simulink model "StabilityObserverPosition"  (R2016b)
settings: configuration reference "WheelSimConfiguration2016" (kept outside this file)
undefined symbols (not defined in the file): simulator
settings Model: Creator=At  LastModifiedBy=At
settings ConfigSetRef: SourceLocation=Base Workspace

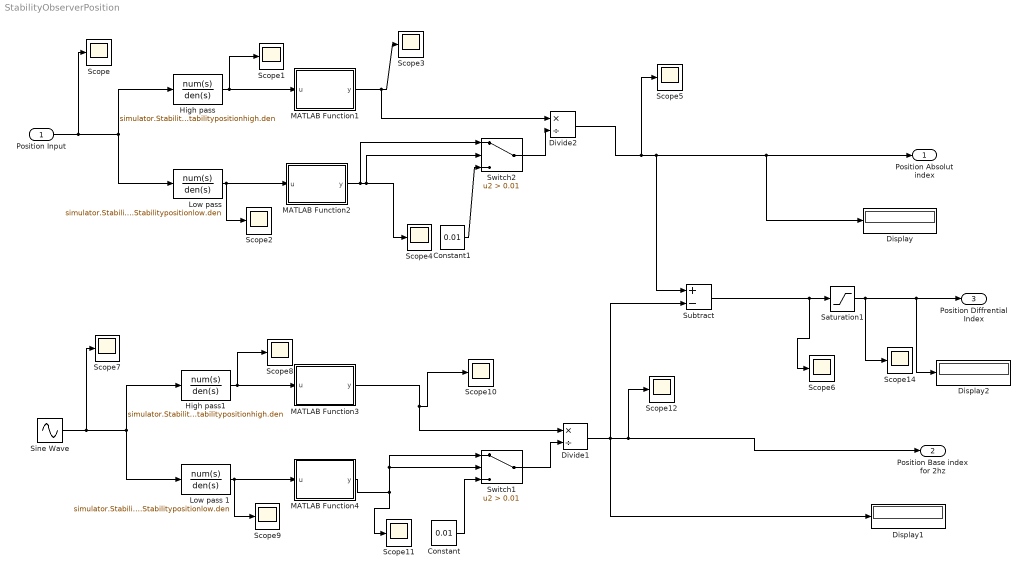
== system StabilityObserverPosition ==
  Position Input : Inport
  Constant : Constant  Value=0.01
  Constant1 : Constant  Value=0.01
  Display : Display
  Display1 : Display
  Display2 : Display
  Divide1 : Product  Inputs=*/
  Divide2 : Product  Inputs=*/
  High pass : TransferFcn  Numerator=simulator.Stabilitypositionhigh.num  Denominator=simulator.Stabilitypositionhigh.den
  High pass1 : TransferFcn  Numerator=simulator.Stabilitypositionhigh.num  Denominator=simulator.Stabilitypositionhigh.den
  "Low pass " : TransferFcn  Numerator=simulator.Stabilitypositionlow.num  Denominator=simulator.Stabilitypositionlow.den
  Low pass 1 : TransferFcn  Numerator=simulator.Stabilitypositionlow.num  Denominator=simulator.Stabilitypositionlow.den
  MATLAB Function1 : MATLAB Function  TreatAsAtomicUnit=on
  MATLAB Function2 : MATLAB Function  TreatAsAtomicUnit=on
  MATLAB Function3 : MATLAB Function  TreatAsAtomicUnit=on
  MATLAB Function4 : MATLAB Function  TreatAsAtomicUnit=on
  Saturation1 : Saturate  UpperLimit=1  LowerLimit=0
  Scope{,1..12,14} (14 alike) : Scope
  Sine Wave : Sin  Amplitude=20  Frequency=2*2*pi  SampleTime=0
  Subtract : Sum  Inputs=+-
  Switch1 : Switch  Criteria=u2 > Threshold  Threshold=0.01
  Switch2 : Switch  Criteria=u2 > Threshold  Threshold=0.01
  Position Absolut index : Outport
  Position Base index for 2hz : Outport  Port=2
  Position Diffrential Index : Outport  Port=3
  wires:
  Position Input/1 -> Scope/1, High pass/1, "Low pass "/1
  High pass/1 -> Scope1/1, MATLAB Function1/1(u)
  "Low pass "/1 -> MATLAB Function2/1(u), Scope2/1
  MATLAB Function2/1(y) -> Switch2/1, Switch2/2, Scope4/1
  Divide2/1 -> Scope5/1, Display/1, Position Absolut index/1, Subtract/1
  Sine Wave/1 -> Scope7/1, High pass1/1, Low pass 1/1
  High pass1/1 -> MATLAB Function3/1(u), Scope8/1
  Low pass 1/1 -> MATLAB Function4/1(u), Scope9/1
  MATLAB Function3/1(y) -> Divide1/1, Scope10/1
  MATLAB Function4/1(y) -> Scope11/1, Switch1/1, Switch1/2
  Constant/1 -> Switch1/3
  Switch1/1 -> Divide1/2
  Saturation1/1 -> Scope14/1, Display2/1, Position Diffrential Index/1
  Subtract/1 -> Scope6/1, Saturation1/1
  Divide1/1 -> Scope12/1, Position Base index for 2hz/1, Display1/1, Subtract/2
  MATLAB Function1/1(y) -> Divide2/1, Scope3/1
  Constant1/1 -> Switch2/3
  Switch2/1 -> Divide2/2

== matlab function StabilityObserverPosition/MATLAB Function1 ==
  data: u input; y output
function y = fcn(u)

y = norm(u);

== matlab function StabilityObserverPosition/MATLAB Function2 ==
  data: u input; y output
function y = fcn(u)

y = norm(u);

== matlab function StabilityObserverPosition/MATLAB Function3 ==
  data: u input; y output
function y = fcn(u)

y = norm(u);

== matlab function StabilityObserverPosition/MATLAB Function4 ==
  data: u input; y output
function y = fcn(u)

y = norm(u);
